simulink model "hybrid_new_eq_circuit_pascal5_single_shot_stack"  (R2019a)
settings: Solver=FixedStepAuto  StartTime=0.0  StopTime=sim_time  FixedStep=resolution  MinStep=0.001  RelTol=1e-4  EnableMultiTasking=on
values from neighbouring files (symbols this model uses):
  amps_in = double(amps_in)    [ClassHybrid.m]    (also in Sc.m = double(amps_in_); workspace_test_model.mat = 0)
  resolution = double(resolution)    [ClassHybrid.m]    (also in Sc.m = double(resolution_); matlab.mat = 1; model_out_all.mat = 0.5; testHyb.m = 0.5)
  tStep = resolution    (= 0.1)    [ClassHybrid.m]    (also in Sc.m; matlab.mat = 10; model_out_all.mat = 1; raw.mat = 1)
libraries: powerlib x525, simulink x9
(part 5 of 8)

== system hybrid_new_eq_circuit_pascal5_single_shot_stack/Battery 2/Subsystem/Subsystem3 ==
  note: Export user input data
  v_r_in : Inport
  v_cap_in : Inport  Port=2
  i_leak_in : Inport  Port=3
  p_chg_in : Inport  Port=4
  p_leak_in : Inport  Port=5
  i_in : Inport  Port=6
  c_in : Inport  Port=7
  r_in : Inport  Port=8
  r_leak_in : Inport  Port=9
  l_in : Inport  Port=10
  Constant : Constant  Value=c
  Constant4 : Constant  Value=r_esr
  Constant5 : Constant  Value=r_leak
  Fcn1 : Fcn  Expr=u^2/r_leak
  Mux{,1..9} (10 alike) : Mux  Inputs=2
  Parallel RLC Branch1 : powerlib/Elements/Parallel RLC Branch  LConnTagsString=a  RConnTagsString=__new0  BranchType=R  Resistance=r_leak  Inductance=1e-3  SetiL0=off  InitialCurrent=0  Capacitance=1e-6  Setx0=off  InitialVoltage=0  Measurements=None
      settings: SourceProductName=Simscape Electrical
  Parallel RLC Branch10 : powerlib/Elements/Parallel RLC Branch  LConnTagsString=a  RConnTagsString=__new0  BranchType=R  Resistance=r_esr  Inductance=1e-3  SetiL0=off  InitialCurrent=0  Capacitance=1e-6  Setx0=off  InitialVoltage=0  Measurements=None
      settings: SourceProductName=Simscape Electrical
  Parallel RLC Branch11 : powerlib/Elements/Parallel RLC Branch  LConnTagsString=a  RConnTagsString=__new0  BranchType=C  Resistance=1  Inductance=1e-3  SetiL0=off  InitialCurrent=0  Capacitance=c  Setx0=on  InitialVoltage=v_init  Measurements=None
      settings: SourceProductName=Simscape Electrical
  i : powerlib/Measurements/Current Measurement  PhasorSimulation=off  OutputType=Complex  PSBequivalent=0
      settings: SourceProductName=Simscape Electrical
  i_leak : powerlib/Measurements/Current Measurement  PhasorSimulation=off  OutputType=Complex  PSBequivalent=0
      settings: SourceProductName=Simscape Electrical
  v^2/R : Fcn  Expr=u^2/r_esr
  v_cap : powerlib/Measurements/Voltage Measurement  PhasorSimulation=off  OutputType=Magnitude  PSBequivalent=0
      settings: SourceProductName=Simscape Electrical
  v_r : powerlib/Measurements/Voltage Measurement  PhasorSimulation=off  OutputType=Complex  PSBequivalent=0
      settings: SourceProductName=Simscape Electrical
  VCC_in : PMIOPort  Side=Left
  VSS_in : PMIOPort  Port=2  Side=Left
  VCC_out : PMIOPort  Tag=PMCPort  Port=3  Side=Right
  VSS_out : PMIOPort  Tag=PMCPort  Port=4  Side=Right
  v_r_out : Outport
  v_cap_out : Outport  Port=2
  i_leak_out : Outport  Port=3
  p_chg_out : Outport  Port=4
  p_leak_out : Outport  Port=5
  i_out : Outport  Port=6
  c_out : Outport  Port=7
  r_out : Outport  Port=8
  r_leak_out : Outport  Port=9
  l_out : Outport  Port=10
  wires:
  i_leak/1 -> Mux2/1
  v_r/1 -> Mux1/1, v^2/R/1
  Mux6/1 -> c_out/1
  Mux7/1 -> r_out/1
  Mux8/1 -> r_leak_out/1
  Mux9/1 -> l_out/1
  Constant/1 -> Mux6/1
  Constant4/1 -> Mux7/1
  Constant5/1 -> Mux8/1
  ? -> Mux9/1
  c_in/1 -> Mux6/2
  l_in/1 -> Mux9/2
  r_leak_in/1 -> Mux8/2
  r_in/1 -> Mux7/2
  p_chg_in/1 -> Mux3/2
  Mux3/1 -> p_chg_out/1
  v_r_in/1 -> Mux1/2
  Mux1/1 -> v_r_out/1
  v^2/R/1 -> Mux3/1
  Mux2/1 -> i_leak_out/1
  i_leak_in/1 -> Mux2/2
  i/1 -> Mux5/1
  Mux5/1 -> i_out/1
  i_in/1 -> Mux5/2
  p_leak_in/1 -> Mux4/2
  Mux4/1 -> p_leak_out/1
  Mux/1 -> v_cap_out/1
  v_cap_in/1 -> Mux/2
  Fcn1/1 -> Mux4/1
  v_cap/1 -> Fcn1/1, Mux/1  "v_cap_out"
  connections:
  Parallel RLC Branch1/RConn1 -- i_leak/LConn1
  VSS_out/RConn1 -- VSS_in/RConn1 -- i_leak/RConn1 -- Parallel RLC Branch11/RConn1 -- v_cap/LConn2
  v_cap/LConn1 -- i/RConn1 -- Parallel RLC Branch11/LConn1 -- Parallel RLC Branch1/LConn1
  VCC_out/RConn1 -- v_r/LConn1 -- Parallel RLC Branch10/LConn1 -- VCC_in/RConn1
  v_r/LConn2 -- i/LConn1 -- Parallel RLC Branch10/RConn1

== system hybrid_new_eq_circuit_pascal5_single_shot_stack/Battery 2/Subsystem/Subsystem5 ==
  note: Export user input data
  v_r_in : Inport
  v_cap_in : Inport  Port=2
  i_leak_in : Inport  Port=3
  p_chg_in : Inport  Port=4
  p_leak_in : Inport  Port=5
  i_in : Inport  Port=6
  c_in : Inport  Port=7
  r_in : Inport  Port=8
  r_leak_in : Inport  Port=9
  l_in : Inport  Port=10
  Constant : Constant  Value=c
  Constant4 : Constant  Value=r_esr
  Constant5 : Constant  Value=r_leak
  Fcn1 : Fcn  Expr=u^2/r_leak
  Mux{,1..9} (10 alike) : Mux  Inputs=2
  Parallel RLC Branch1 : powerlib/Elements/Parallel RLC Branch  LConnTagsString=a  RConnTagsString=__new0  BranchType=R  Resistance=r_leak  Inductance=1e-3  SetiL0=off  InitialCurrent=0  Capacitance=1e-6  Setx0=off  InitialVoltage=0  Measurements=None
      settings: SourceProductName=Simscape Electrical
  Parallel RLC Branch10 : powerlib/Elements/Parallel RLC Branch  LConnTagsString=a  RConnTagsString=__new0  BranchType=R  Resistance=r_esr  Inductance=1e-3  SetiL0=off  InitialCurrent=0  Capacitance=1e-6  Setx0=off  InitialVoltage=0  Measurements=None
      settings: SourceProductName=Simscape Electrical
  Parallel RLC Branch11 : powerlib/Elements/Parallel RLC Branch  LConnTagsString=a  RConnTagsString=__new0  BranchType=C  Resistance=1  Inductance=1e-3  SetiL0=off  InitialCurrent=0  Capacitance=c  Setx0=on  InitialVoltage=v_init  Measurements=None
      settings: SourceProductName=Simscape Electrical
  i : powerlib/Measurements/Current Measurement  PhasorSimulation=off  OutputType=Complex  PSBequivalent=0
      settings: SourceProductName=Simscape Electrical
  i_leak : powerlib/Measurements/Current Measurement  PhasorSimulation=off  OutputType=Complex  PSBequivalent=0
      settings: SourceProductName=Simscape Electrical
  v^2/R : Fcn  Expr=u^2/r_esr
  v_cap : powerlib/Measurements/Voltage Measurement  PhasorSimulation=off  OutputType=Magnitude  PSBequivalent=0
      settings: SourceProductName=Simscape Electrical
  v_r : powerlib/Measurements/Voltage Measurement  PhasorSimulation=off  OutputType=Complex  PSBequivalent=0
      settings: SourceProductName=Simscape Electrical
  VCC_in : PMIOPort  Side=Left
  VSS_in : PMIOPort  Port=2  Side=Left
  VCC_out : PMIOPort  Tag=PMCPort  Port=3  Side=Right
  VSS_out : PMIOPort  Tag=PMCPort  Port=4  Side=Right
  v_r_out : Outport
  v_cap_out : Outport  Port=2
  i_leak_out : Outport  Port=3
  p_chg_out : Outport  Port=4
  p_leak_out : Outport  Port=5
  i_out : Outport  Port=6
  c_out : Outport  Port=7
  r_out : Outport  Port=8
  r_leak_out : Outport  Port=9
  l_out : Outport  Port=10
  wires:
  Fcn1/1 -> Mux4/1
  v_cap_in/1 -> Mux/2
  Mux/1 -> v_cap_out/1
  Mux4/1 -> p_leak_out/1
  p_leak_in/1 -> Mux4/2
  i_in/1 -> Mux5/2
  Mux5/1 -> i_out/1
  i/1 -> Mux5/1
  i_leak_in/1 -> Mux2/2
  Mux2/1 -> i_leak_out/1
  v^2/R/1 -> Mux3/1
  Mux1/1 -> v_r_out/1
  v_r_in/1 -> Mux1/2
  Mux3/1 -> p_chg_out/1
  p_chg_in/1 -> Mux3/2
  r_in/1 -> Mux7/2
  r_leak_in/1 -> Mux8/2
  l_in/1 -> Mux9/2
  c_in/1 -> Mux6/2
  ? -> Mux9/1
  Constant5/1 -> Mux8/1
  Constant4/1 -> Mux7/1
  Constant/1 -> Mux6/1
  Mux9/1 -> l_out/1
  Mux8/1 -> r_leak_out/1
  Mux7/1 -> r_out/1
  Mux6/1 -> c_out/1
  v_r/1 -> v^2/R/1, Mux1/1
  i_leak/1 -> Mux2/1
  v_cap/1 -> Fcn1/1, Mux/1  "v_cap_out"
  connections:
  Parallel RLC Branch10/RConn1 -- i/LConn1 -- v_r/LConn2
  VCC_in/RConn1 -- Parallel RLC Branch10/LConn1 -- v_r/LConn1 -- VCC_out/RConn1
  Parallel RLC Branch11/LConn1 -- i/RConn1 -- Parallel RLC Branch1/LConn1 -- v_cap/LConn1
  v_cap/LConn2 -- Parallel RLC Branch11/RConn1 -- i_leak/RConn1 -- VSS_in/RConn1 -- VSS_out/RConn1
  Parallel RLC Branch1/RConn1 -- i_leak/LConn1

== system hybrid_new_eq_circuit_pascal5_single_shot_stack/Battery 3/Subsystem/Subsystem1 ==
  note: Export user input data
  v_r_in : Inport
  v_cap_in : Inport  Port=2
  i_leak_in : Inport  Port=3
  p_chg_in : Inport  Port=4
  p_leak_in : Inport  Port=5
  i_in : Inport  Port=6
  c_in : Inport  Port=7
  r_in : Inport  Port=8
  r_leak_in : Inport  Port=9
  l_in : Inport  Port=10
  Constant : Constant  Value=c
  Constant4 : Constant  Value=r_esr
  Constant5 : Constant  Value=r_leak
  Fcn1 : Fcn  Expr=u^2/r_leak
  Mux{,1..9} (10 alike) : Mux  Inputs=2
  Parallel RLC Branch1 : powerlib/Elements/Parallel RLC Branch  LConnTagsString=a  RConnTagsString=__new0  BranchType=R  Resistance=r_leak  Inductance=1e-3  SetiL0=off  InitialCurrent=0  Capacitance=1e-6  Setx0=off  InitialVoltage=0  Measurements=None
      settings: SourceProductName=Simscape Electrical
  Parallel RLC Branch10 : powerlib/Elements/Parallel RLC Branch  LConnTagsString=a  RConnTagsString=__new0  BranchType=R  Resistance=r_esr  Inductance=1e-3  SetiL0=off  InitialCurrent=0  Capacitance=1e-6  Setx0=off  InitialVoltage=0  Measurements=None
      settings: SourceProductName=Simscape Electrical
  Parallel RLC Branch11 : powerlib/Elements/Parallel RLC Branch  LConnTagsString=a  RConnTagsString=__new0  BranchType=C  Resistance=1  Inductance=1e-3  SetiL0=off  InitialCurrent=0  Capacitance=c  Setx0=on  InitialVoltage=v_init  Measurements=None
      settings: SourceProductName=Simscape Electrical
  i : powerlib/Measurements/Current Measurement  PhasorSimulation=off  OutputType=Complex  PSBequivalent=0
      settings: SourceProductName=Simscape Electrical
  i_leak : powerlib/Measurements/Current Measurement  PhasorSimulation=off  OutputType=Complex  PSBequivalent=0
      settings: SourceProductName=Simscape Electrical
  v^2/R : Fcn  Expr=u^2/r_esr
  v_cap : powerlib/Measurements/Voltage Measurement  PhasorSimulation=off  OutputType=Magnitude  PSBequivalent=0
      settings: SourceProductName=Simscape Electrical
  v_r : powerlib/Measurements/Voltage Measurement  PhasorSimulation=off  OutputType=Complex  PSBequivalent=0
      settings: SourceProductName=Simscape Electrical
  VCC_in : PMIOPort  Side=Left
  VSS_in : PMIOPort  Port=2  Side=Left
  VCC_out : PMIOPort  Tag=PMCPort  Port=3  Side=Right
  VSS_out : PMIOPort  Tag=PMCPort  Port=4  Side=Right
  v_r_out : Outport
  v_cap_out : Outport  Port=2
  i_leak_out : Outport  Port=3
  p_chg_out : Outport  Port=4
  p_leak_out : Outport  Port=5
  i_out : Outport  Port=6
  c_out : Outport  Port=7
  r_out : Outport  Port=8
  r_leak_out : Outport  Port=9
  l_out : Outport  Port=10
  wires:
  i_leak/1 -> Mux2/1
  v_r/1 -> Mux1/1, v^2/R/1
  Mux6/1 -> c_out/1
  Mux7/1 -> r_out/1
  Mux8/1 -> r_leak_out/1
  Mux9/1 -> l_out/1
  Constant/1 -> Mux6/1
  Constant4/1 -> Mux7/1
  Constant5/1 -> Mux8/1
  ? -> Mux9/1
  c_in/1 -> Mux6/2
  l_in/1 -> Mux9/2
  r_leak_in/1 -> Mux8/2
  r_in/1 -> Mux7/2
  p_chg_in/1 -> Mux3/2
  Mux3/1 -> p_chg_out/1
  v_r_in/1 -> Mux1/2
  Mux1/1 -> v_r_out/1
  v^2/R/1 -> Mux3/1
  Mux2/1 -> i_leak_out/1
  i_leak_in/1 -> Mux2/2
  i/1 -> Mux5/1
  Mux5/1 -> i_out/1
  i_in/1 -> Mux5/2
  p_leak_in/1 -> Mux4/2
  Mux4/1 -> p_leak_out/1
  Mux/1 -> v_cap_out/1
  v_cap_in/1 -> Mux/2
  Fcn1/1 -> Mux4/1
  v_cap/1 -> Fcn1/1, Mux/1  "v_cap_out"
  connections:
  Parallel RLC Branch1/RConn1 -- i_leak/LConn1
  VSS_out/RConn1 -- VSS_in/RConn1 -- i_leak/RConn1 -- Parallel RLC Branch11/RConn1 -- v_cap/LConn2
  v_cap/LConn1 -- i/RConn1 -- Parallel RLC Branch11/LConn1 -- Parallel RLC Branch1/LConn1
  VCC_out/RConn1 -- v_r/LConn1 -- Parallel RLC Branch10/LConn1 -- VCC_in/RConn1
  v_r/LConn2 -- i/LConn1 -- Parallel RLC Branch10/RConn1

== system hybrid_new_eq_circuit_pascal5_single_shot_stack/Battery 3/Subsystem/Subsystem2 ==
  note: Export user input data
  v_r_in : Inport
  v_cap_in : Inport  Port=2
  i_leak_in : Inport  Port=3
  p_chg_in : Inport  Port=4
  p_leak_in : Inport  Port=5
  i_in : Inport  Port=6
  c_in : Inport  Port=7
  r_in : Inport  Port=8
  r_leak_in : Inport  Port=9
  l_in : Inport  Port=10
  Constant : Constant  Value=c
  Constant4 : Constant  Value=r_esr
  Constant5 : Constant  Value=r_leak
  Fcn1 : Fcn  Expr=u^2/r_leak
  Mux{,1..9} (10 alike) : Mux  Inputs=2
  Parallel RLC Branch1 : powerlib/Elements/Parallel RLC Branch  LConnTagsString=a  RConnTagsString=__new0  BranchType=R  Resistance=r_leak  Inductance=1e-3  SetiL0=off  InitialCurrent=0  Capacitance=1e-6  Setx0=off  InitialVoltage=0  Measurements=None
      settings: SourceProductName=Simscape Electrical
  Parallel RLC Branch10 : powerlib/Elements/Parallel RLC Branch  LConnTagsString=a  RConnTagsString=__new0  BranchType=R  Resistance=r_esr  Inductance=1e-3  SetiL0=off  InitialCurrent=0  Capacitance=1e-6  Setx0=off  InitialVoltage=0  Measurements=None
      settings: SourceProductName=Simscape Electrical
  Parallel RLC Branch11 : powerlib/Elements/Parallel RLC Branch  LConnTagsString=a  RConnTagsString=__new0  BranchType=C  Resistance=1  Inductance=1e-3  SetiL0=off  InitialCurrent=0  Capacitance=c  Setx0=on  InitialVoltage=v_init  Measurements=None
      settings: SourceProductName=Simscape Electrical
  i : powerlib/Measurements/Current Measurement  PhasorSimulation=off  OutputType=Complex  PSBequivalent=0
      settings: SourceProductName=Simscape Electrical
  i_leak : powerlib/Measurements/Current Measurement  PhasorSimulation=off  OutputType=Complex  PSBequivalent=0
      settings: SourceProductName=Simscape Electrical
  v^2/R : Fcn  Expr=u^2/r_esr
  v_cap : powerlib/Measurements/Voltage Measurement  PhasorSimulation=off  OutputType=Magnitude  PSBequivalent=0
      settings: SourceProductName=Simscape Electrical
  v_r : powerlib/Measurements/Voltage Measurement  PhasorSimulation=off  OutputType=Complex  PSBequivalent=0
      settings: SourceProductName=Simscape Electrical
  VCC_in : PMIOPort  Side=Left
  VSS_in : PMIOPort  Port=2  Side=Left
  VCC_out : PMIOPort  Tag=PMCPort  Port=3  Side=Right
  VSS_out : PMIOPort  Tag=PMCPort  Port=4  Side=Right
  v_r_out : Outport
  v_cap_out : Outport  Port=2
  i_leak_out : Outport  Port=3
  p_chg_out : Outport  Port=4
  p_leak_out : Outport  Port=5
  i_out : Outport  Port=6
  c_out : Outport  Port=7
  r_out : Outport  Port=8
  r_leak_out : Outport  Port=9
  l_out : Outport  Port=10
  wires:
  Fcn1/1 -> Mux4/1
  v_cap_in/1 -> Mux/2
  Mux/1 -> v_cap_out/1
  Mux4/1 -> p_leak_out/1
  p_leak_in/1 -> Mux4/2
  i_in/1 -> Mux5/2
  Mux5/1 -> i_out/1
  i/1 -> Mux5/1
  i_leak_in/1 -> Mux2/2
  Mux2/1 -> i_leak_out/1
  v^2/R/1 -> Mux3/1
  Mux1/1 -> v_r_out/1
  v_r_in/1 -> Mux1/2
  Mux3/1 -> p_chg_out/1
  p_chg_in/1 -> Mux3/2
  r_in/1 -> Mux7/2
  r_leak_in/1 -> Mux8/2
  l_in/1 -> Mux9/2
  c_in/1 -> Mux6/2
  ? -> Mux9/1
  Constant5/1 -> Mux8/1
  Constant4/1 -> Mux7/1
  Constant/1 -> Mux6/1
  Mux9/1 -> l_out/1
  Mux8/1 -> r_leak_out/1
  Mux7/1 -> r_out/1
  Mux6/1 -> c_out/1
  v_r/1 -> v^2/R/1, Mux1/1
  i_leak/1 -> Mux2/1
  v_cap/1 -> Mux/1, Fcn1/1  "v_cap_out"
  connections:
  Parallel RLC Branch10/RConn1 -- i/LConn1 -- v_r/LConn2
  VCC_in/RConn1 -- Parallel RLC Branch10/LConn1 -- v_r/LConn1 -- VCC_out/RConn1
  Parallel RLC Branch1/LConn1 -- Parallel RLC Branch11/LConn1 -- i/RConn1 -- v_cap/LConn1
  v_cap/LConn2 -- Parallel RLC Branch11/RConn1 -- i_leak/RConn1 -- VSS_in/RConn1 -- VSS_out/RConn1
  Parallel RLC Branch1/RConn1 -- i_leak/LConn1

== system hybrid_new_eq_circuit_pascal5_single_shot_stack/Battery 3/Subsystem/Subsystem3 ==
  note: Export user input data
  v_r_in : Inport
  v_cap_in : Inport  Port=2
  i_leak_in : Inport  Port=3
  p_chg_in : Inport  Port=4
  p_leak_in : Inport  Port=5
  i_in : Inport  Port=6
  c_in : Inport  Port=7
  r_in : Inport  Port=8
  r_leak_in : Inport  Port=9
  l_in : Inport  Port=10
  Constant : Constant  Value=c
  Constant4 : Constant  Value=r_esr
  Constant5 : Constant  Value=r_leak
  Fcn1 : Fcn  Expr=u^2/r_leak
  Mux{,1..9} (10 alike) : Mux  Inputs=2
  Parallel RLC Branch1 : powerlib/Elements/Parallel RLC Branch  LConnTagsString=a  RConnTagsString=__new0  BranchType=R  Resistance=r_leak  Inductance=1e-3  SetiL0=off  InitialCurrent=0  Capacitance=1e-6  Setx0=off  InitialVoltage=0  Measurements=None
      settings: SourceProductName=Simscape Electrical
  Parallel RLC Branch10 : powerlib/Elements/Parallel RLC Branch  LConnTagsString=a  RConnTagsString=__new0  BranchType=R  Resistance=r_esr  Inductance=1e-3  SetiL0=off  InitialCurrent=0  Capacitance=1e-6  Setx0=off  InitialVoltage=0  Measurements=None
      settings: SourceProductName=Simscape Electrical
  Parallel RLC Branch11 : powerlib/Elements/Parallel RLC Branch  LConnTagsString=a  RConnTagsString=__new0  BranchType=C  Resistance=1  Inductance=1e-3  SetiL0=off  InitialCurrent=0  Capacitance=c  Setx0=on  InitialVoltage=v_init  Measurements=None
      settings: SourceProductName=Simscape Electrical
  i : powerlib/Measurements/Current Measurement  PhasorSimulation=off  OutputType=Complex  PSBequivalent=0
      settings: SourceProductName=Simscape Electrical
  i_leak : powerlib/Measurements/Current Measurement  PhasorSimulation=off  OutputType=Complex  PSBequivalent=0
      settings: SourceProductName=Simscape Electrical
  v^2/R : Fcn  Expr=u^2/r_esr
  v_cap : powerlib/Measurements/Voltage Measurement  PhasorSimulation=off  OutputType=Magnitude  PSBequivalent=0
      settings: SourceProductName=Simscape Electrical
  v_r : powerlib/Measurements/Voltage Measurement  PhasorSimulation=off  OutputType=Complex  PSBequivalent=0
      settings: SourceProductName=Simscape Electrical
  VCC_in : PMIOPort  Side=Left
  VSS_in : PMIOPort  Port=2  Side=Left
  VCC_out : PMIOPort  Tag=PMCPort  Port=3  Side=Right
  VSS_out : PMIOPort  Tag=PMCPort  Port=4  Side=Right
  v_r_out : Outport
  v_cap_out : Outport  Port=2
  i_leak_out : Outport  Port=3
  p_chg_out : Outport  Port=4
  p_leak_out : Outport  Port=5
  i_out : Outport  Port=6
  c_out : Outport  Port=7
  r_out : Outport  Port=8
  r_leak_out : Outport  Port=9
  l_out : Outport  Port=10
  wires:
  i_leak/1 -> Mux2/1
  v_r/1 -> Mux1/1, v^2/R/1
  Mux6/1 -> c_out/1
  Mux7/1 -> r_out/1
  Mux8/1 -> r_leak_out/1
  Mux9/1 -> l_out/1
  Constant/1 -> Mux6/1
  Constant4/1 -> Mux7/1
  Constant5/1 -> Mux8/1
  ? -> Mux9/1
  c_in/1 -> Mux6/2
  l_in/1 -> Mux9/2
  r_leak_in/1 -> Mux8/2
  r_in/1 -> Mux7/2
  p_chg_in/1 -> Mux3/2
  Mux3/1 -> p_chg_out/1
  v_r_in/1 -> Mux1/2
  Mux1/1 -> v_r_out/1
  v^2/R/1 -> Mux3/1
  Mux2/1 -> i_leak_out/1
  i_leak_in/1 -> Mux2/2
  i/1 -> Mux5/1
  Mux5/1 -> i_out/1
  i_in/1 -> Mux5/2
  p_leak_in/1 -> Mux4/2
  Mux4/1 -> p_leak_out/1
  Mux/1 -> v_cap_out/1
  v_cap_in/1 -> Mux/2
  Fcn1/1 -> Mux4/1
  v_cap/1 -> Fcn1/1, Mux/1  "v_cap_out"
  connections:
  Parallel RLC Branch1/RConn1 -- i_leak/LConn1
  VSS_out/RConn1 -- VSS_in/RConn1 -- i_leak/RConn1 -- Parallel RLC Branch11/RConn1 -- v_cap/LConn2
  v_cap/LConn1 -- i/RConn1 -- Parallel RLC Branch11/LConn1 -- Parallel RLC Branch1/LConn1
  VCC_out/RConn1 -- v_r/LConn1 -- Parallel RLC Branch10/LConn1 -- VCC_in/RConn1
  v_r/LConn2 -- i/LConn1 -- Parallel RLC Branch10/RConn1

== system hybrid_new_eq_circuit_pascal5_single_shot_stack/Battery 3/Subsystem/Subsystem5 ==
  note: Export user input data
  v_r_in : Inport
  v_cap_in : Inport  Port=2
  i_leak_in : Inport  Port=3
  p_chg_in : Inport  Port=4
  p_leak_in : Inport  Port=5
  i_in : Inport  Port=6
  c_in : Inport  Port=7
  r_in : Inport  Port=8
  r_leak_in : Inport  Port=9
  l_in : Inport  Port=10
  Constant : Constant  Value=c
  Constant4 : Constant  Value=r_esr
  Constant5 : Constant  Value=r_leak
  Fcn1 : Fcn  Expr=u^2/r_leak
  Mux{,1..9} (10 alike) : Mux  Inputs=2
  Parallel RLC Branch1 : powerlib/Elements/Parallel RLC Branch  LConnTagsString=a  RConnTagsString=__new0  BranchType=R  Resistance=r_leak  Inductance=1e-3  SetiL0=off  InitialCurrent=0  Capacitance=1e-6  Setx0=off  InitialVoltage=0  Measurements=None
      settings: SourceProductName=Simscape Electrical
  Parallel RLC Branch10 : powerlib/Elements/Parallel RLC Branch  LConnTagsString=a  RConnTagsString=__new0  BranchType=R  Resistance=r_esr  Inductance=1e-3  SetiL0=off  InitialCurrent=0  Capacitance=1e-6  Setx0=off  InitialVoltage=0  Measurements=None
      settings: SourceProductName=Simscape Electrical
  Parallel RLC Branch11 : powerlib/Elements/Parallel RLC Branch  LConnTagsString=a  RConnTagsString=__new0  BranchType=C  Resistance=1  Inductance=1e-3  SetiL0=off  InitialCurrent=0  Capacitance=c  Setx0=on  InitialVoltage=v_init  Measurements=None
      settings: SourceProductName=Simscape Electrical
  i : powerlib/Measurements/Current Measurement  PhasorSimulation=off  OutputType=Complex  PSBequivalent=0
      settings: SourceProductName=Simscape Electrical
  i_leak : powerlib/Measurements/Current Measurement  PhasorSimulation=off  OutputType=Complex  PSBequivalent=0
      settings: SourceProductName=Simscape Electrical
  v^2/R : Fcn  Expr=u^2/r_esr
  v_cap : powerlib/Measurements/Voltage Measurement  PhasorSimulation=off  OutputType=Magnitude  PSBequivalent=0
      settings: SourceProductName=Simscape Electrical
  v_r : powerlib/Measurements/Voltage Measurement  PhasorSimulation=off  OutputType=Complex  PSBequivalent=0
      settings: SourceProductName=Simscape Electrical
  VCC_in : PMIOPort  Side=Left
  VSS_in : PMIOPort  Port=2  Side=Left
  VCC_out : PMIOPort  Tag=PMCPort  Port=3  Side=Right
  VSS_out : PMIOPort  Tag=PMCPort  Port=4  Side=Right
  v_r_out : Outport
  v_cap_out : Outport  Port=2
  i_leak_out : Outport  Port=3
  p_chg_out : Outport  Port=4
  p_leak_out : Outport  Port=5
  i_out : Outport  Port=6
  c_out : Outport  Port=7
  r_out : Outport  Port=8
  r_leak_out : Outport  Port=9
  l_out : Outport  Port=10
  wires:
  Fcn1/1 -> Mux4/1
  v_cap_in/1 -> Mux/2
  Mux/1 -> v_cap_out/1
  Mux4/1 -> p_leak_out/1
  p_leak_in/1 -> Mux4/2
  i_in/1 -> Mux5/2
  Mux5/1 -> i_out/1
  i/1 -> Mux5/1
  i_leak_in/1 -> Mux2/2
  Mux2/1 -> i_leak_out/1
  v^2/R/1 -> Mux3/1
  Mux1/1 -> v_r_out/1
  v_r_in/1 -> Mux1/2
  Mux3/1 -> p_chg_out/1
  p_chg_in/1 -> Mux3/2
  r_in/1 -> Mux7/2
  r_leak_in/1 -> Mux8/2
  l_in/1 -> Mux9/2
  c_in/1 -> Mux6/2
  ? -> Mux9/1
  Constant5/1 -> Mux8/1
  Constant4/1 -> Mux7/1
  Constant/1 -> Mux6/1
  Mux9/1 -> l_out/1
  Mux8/1 -> r_leak_out/1
  Mux7/1 -> r_out/1
  Mux6/1 -> c_out/1
  v_r/1 -> v^2/R/1, Mux1/1
  i_leak/1 -> Mux2/1
  v_cap/1 -> Fcn1/1, Mux/1  "v_cap_out"
  connections:
  Parallel RLC Branch10/RConn1 -- i/LConn1 -- v_r/LConn2
  VCC_in/RConn1 -- Parallel RLC Branch10/LConn1 -- v_r/LConn1 -- VCC_out/RConn1
  Parallel RLC Branch11/LConn1 -- i/RConn1 -- Parallel RLC Branch1/LConn1 -- v_cap/LConn1
  v_cap/LConn2 -- Parallel RLC Branch11/RConn1 -- i_leak/RConn1 -- VSS_in/RConn1 -- VSS_out/RConn1
  Parallel RLC Branch1/RConn1 -- i_leak/LConn1

== system hybrid_new_eq_circuit_pascal5_single_shot_stack/Supercapacitor 1/Subsystem/Subsystem1 ==
  note: Export user input data
  v_r_in : Inport
  v_cap_in : Inport  Port=2
  i_leak_in : Inport  Port=3
  p_chg_in : Inport  Port=4
  p_leak_in : Inport  Port=5
  i_in : Inport  Port=6
  c_in : Inport  Port=7
  r_in : Inport  Port=8
  r_leak_in : Inport  Port=9
  l_in : Inport  Port=10
  Constant : Constant  Value=c
  Constant4 : Constant  Value=r_esr
  Constant5 : Constant  Value=r_leak
  Fcn1 : Fcn  Expr=u^2/r_leak
  Mux{,1..9} (10 alike) : Mux  Inputs=2
  Parallel RLC Branch1 : powerlib/Elements/Parallel RLC Branch  LConnTagsString=a  RConnTagsString=__new0  BranchType=R  Resistance=r_leak  Inductance=1e-3  SetiL0=off  InitialCurrent=0  Capacitance=1e-6  Setx0=off  InitialVoltage=0  Measurements=None
      settings: SourceProductName=Simscape Electrical
  Parallel RLC Branch10 : powerlib/Elements/Parallel RLC Branch  LConnTagsString=a  RConnTagsString=__new0  BranchType=R  Resistance=r_esr  Inductance=1e-3  SetiL0=off  InitialCurrent=0  Capacitance=1e-6  Setx0=off  InitialVoltage=0  Measurements=None
      settings: SourceProductName=Simscape Electrical
  Parallel RLC Branch11 : powerlib/Elements/Parallel RLC Branch  LConnTagsString=a  RConnTagsString=__new0  BranchType=C  Resistance=1  Inductance=1e-3  SetiL0=off  InitialCurrent=0  Capacitance=c  Setx0=on  InitialVoltage=v_init  Measurements=None
      settings: SourceProductName=Simscape Electrical
  i : powerlib/Measurements/Current Measurement  PhasorSimulation=off  OutputType=Complex  PSBequivalent=0
      settings: SourceProductName=Simscape Electrical
  i_leak : powerlib/Measurements/Current Measurement  PhasorSimulation=off  OutputType=Complex  PSBequivalent=0
      settings: SourceProductName=Simscape Electrical
  v^2/R : Fcn  Expr=u^2/r_esr
  v_cap : powerlib/Measurements/Voltage Measurement  PhasorSimulation=off  OutputType=Complex  PSBequivalent=0
      settings: SourceProductName=Simscape Electrical
  v_r : powerlib/Measurements/Voltage Measurement  PhasorSimulation=off  OutputType=Complex  PSBequivalent=0
      settings: SourceProductName=Simscape Electrical
  VCC_in : PMIOPort  Side=Left
  VSS_in : PMIOPort  Port=2  Side=Left
  VCC_out : PMIOPort  Tag=PMCPort  Port=3  Side=Right
  VSS_out : PMIOPort  Tag=PMCPort  Port=4  Side=Right
  v_r_out : Outport
  v_cap_out : Outport  Port=2
  i_leak_out : Outport  Port=3
  p_chg_out : Outport  Port=4
  p_leak_out : Outport  Port=5
  i_out : Outport  Port=6
  c_out : Outport  Port=7
  r_out : Outport  Port=8
  r_leak_out : Outport  Port=9
  l_out : Outport  Port=10
  wires:
  Fcn1/1 -> Mux4/1
  v_cap/1 -> Mux/1, Fcn1/1
  v_cap_in/1 -> Mux/2
  Mux/1 -> v_cap_out/1
  Mux4/1 -> p_leak_out/1
  p_leak_in/1 -> Mux4/2
  i_in/1 -> Mux5/2
  Mux5/1 -> i_out/1
  i/1 -> Mux5/1
  i_leak_in/1 -> Mux2/2
  Mux2/1 -> i_leak_out/1
  v^2/R/1 -> Mux3/1
  Mux1/1 -> v_r_out/1
  v_r_in/1 -> Mux1/2
  Mux3/1 -> p_chg_out/1
  p_chg_in/1 -> Mux3/2
  r_in/1 -> Mux7/2
  r_leak_in/1 -> Mux8/2
  l_in/1 -> Mux9/2
  c_in/1 -> Mux6/2
  ? -> Mux9/1
  Constant5/1 -> Mux8/1
  Constant4/1 -> Mux7/1
  Constant/1 -> Mux6/1
  Mux9/1 -> l_out/1
  Mux8/1 -> r_leak_out/1
  Mux7/1 -> r_out/1
  Mux6/1 -> c_out/1
  v_r/1 -> v^2/R/1, Mux1/1
  i_leak/1 -> Mux2/1
  connections:
  Parallel RLC Branch10/RConn1 -- i/LConn1 -- v_r/LConn2
  VCC_in/RConn1 -- Parallel RLC Branch10/LConn1 -- v_r/LConn1 -- VCC_out/RConn1
  Parallel RLC Branch1/LConn1 -- Parallel RLC Branch11/LConn1 -- i/RConn1 -- v_cap/LConn1
  v_cap/LConn2 -- Parallel RLC Branch11/RConn1 -- i_leak/RConn1 -- VSS_in/RConn1 -- VSS_out/RConn1
  Parallel RLC Branch1/RConn1 -- i_leak/LConn1

== system hybrid_new_eq_circuit_pascal5_single_shot_stack/Supercapacitor 1/Subsystem/Subsystem2 ==
  note: Export user input data
  v_r_in : Inport
  v_cap_in : Inport  Port=2
  i_leak_in : Inport  Port=3
  p_chg_in : Inport  Port=4
  p_leak_in : Inport  Port=5
  i_in : Inport  Port=6
  c_in : Inport  Port=7
  r_in : Inport  Port=8
  r_leak_in : Inport  Port=9
  l_in : Inport  Port=10
  Constant : Constant  Value=c
  Constant4 : Constant  Value=r_esr
  Constant5 : Constant  Value=r_leak
  Fcn1 : Fcn  Expr=u^2/r_leak
  Mux{,1..9} (10 alike) : Mux  Inputs=2
  Parallel RLC Branch1 : powerlib/Elements/Parallel RLC Branch  LConnTagsString=a  RConnTagsString=__new0  BranchType=R  Resistance=r_leak  Inductance=1e-3  SetiL0=off  InitialCurrent=0  Capacitance=1e-6  Setx0=off  InitialVoltage=0  Measurements=None
      settings: SourceProductName=Simscape Electrical
  Parallel RLC Branch10 : powerlib/Elements/Parallel RLC Branch  LConnTagsString=a  RConnTagsString=__new0  BranchType=R  Resistance=r_esr  Inductance=1e-3  SetiL0=off  InitialCurrent=0  Capacitance=1e-6  Setx0=off  InitialVoltage=0  Measurements=None
      settings: SourceProductName=Simscape Electrical
  Parallel RLC Branch11 : powerlib/Elements/Parallel RLC Branch  LConnTagsString=a  RConnTagsString=__new0  BranchType=C  Resistance=1  Inductance=1e-3  SetiL0=off  InitialCurrent=0  Capacitance=c  Setx0=on  InitialVoltage=v_init  Measurements=None
      settings: SourceProductName=Simscape Electrical
  i : powerlib/Measurements/Current Measurement  PhasorSimulation=off  OutputType=Complex  PSBequivalent=0
      settings: SourceProductName=Simscape Electrical
  i_leak : powerlib/Measurements/Current Measurement  PhasorSimulation=off  OutputType=Complex  PSBequivalent=0
      settings: SourceProductName=Simscape Electrical
  v^2/R : Fcn  Expr=u^2/r_esr
  v_cap : powerlib/Measurements/Voltage Measurement  PhasorSimulation=off  OutputType=Complex  PSBequivalent=0
      settings: SourceProductName=Simscape Electrical
  v_r : powerlib/Measurements/Voltage Measurement  PhasorSimulation=off  OutputType=Complex  PSBequivalent=0
      settings: SourceProductName=Simscape Electrical
  VCC_in : PMIOPort  Side=Left
  VSS_in : PMIOPort  Port=2  Side=Left
  VCC_out : PMIOPort  Tag=PMCPort  Port=3  Side=Right
  VSS_out : PMIOPort  Tag=PMCPort  Port=4  Side=Right
  v_r_out : Outport
  v_cap_out : Outport  Port=2
  i_leak_out : Outport  Port=3
  p_chg_out : Outport  Port=4
  p_leak_out : Outport  Port=5
  i_out : Outport  Port=6
  c_out : Outport  Port=7
  r_out : Outport  Port=8
  r_leak_out : Outport  Port=9
  l_out : Outport  Port=10
  wires:
  i_leak/1 -> Mux2/1
  v_r/1 -> Mux1/1, v^2/R/1
  Mux6/1 -> c_out/1
  Mux7/1 -> r_out/1
  Mux8/1 -> r_leak_out/1
  Mux9/1 -> l_out/1
  Constant/1 -> Mux6/1
  Constant4/1 -> Mux7/1
  Constant5/1 -> Mux8/1
  ? -> Mux9/1
  c_in/1 -> Mux6/2
  l_in/1 -> Mux9/2
  r_leak_in/1 -> Mux8/2
  r_in/1 -> Mux7/2
  p_chg_in/1 -> Mux3/2
  Mux3/1 -> p_chg_out/1
  v_r_in/1 -> Mux1/2
  Mux1/1 -> v_r_out/1
  v^2/R/1 -> Mux3/1
  Mux2/1 -> i_leak_out/1
  i_leak_in/1 -> Mux2/2
  i/1 -> Mux5/1
  Mux5/1 -> i_out/1
  i_in/1 -> Mux5/2
  p_leak_in/1 -> Mux4/2
  Mux4/1 -> p_leak_out/1
  Mux/1 -> v_cap_out/1
  v_cap_in/1 -> Mux/2
  v_cap/1 -> Fcn1/1, Mux/1
  Fcn1/1 -> Mux4/1
  connections:
  Parallel RLC Branch1/RConn1 -- i_leak/LConn1
  VSS_out/RConn1 -- VSS_in/RConn1 -- i_leak/RConn1 -- Parallel RLC Branch11/RConn1 -- v_cap/LConn2
  v_cap/LConn1 -- i/RConn1 -- Parallel RLC Branch11/LConn1 -- Parallel RLC Branch1/LConn1
  VCC_out/RConn1 -- v_r/LConn1 -- Parallel RLC Branch10/LConn1 -- VCC_in/RConn1
  v_r/LConn2 -- i/LConn1 -- Parallel RLC Branch10/RConn1

== system hybrid_new_eq_circuit_pascal5_single_shot_stack/Supercapacitor 1/Subsystem/Subsystem3 ==
  note: Export user input data
  v_r_in : Inport
  v_cap_in : Inport  Port=2
  i_leak_in : Inport  Port=3
  p_chg_in : Inport  Port=4
  p_leak_in : Inport  Port=5
  i_in : Inport  Port=6
  c_in : Inport  Port=7
  r_in : Inport  Port=8
  r_leak_in : Inport  Port=9
  l_in : Inport  Port=10
  Constant : Constant  Value=c
  Constant4 : Constant  Value=r_esr
  Constant5 : Constant  Value=r_leak
  Fcn1 : Fcn  Expr=u^2/r_leak
  Mux{,1..9} (10 alike) : Mux  Inputs=2
  Parallel RLC Branch1 : powerlib/Elements/Parallel RLC Branch  LConnTagsString=a  RConnTagsString=__new0  BranchType=R  Resistance=r_leak  Inductance=1e-3  SetiL0=off  InitialCurrent=0  Capacitance=1e-6  Setx0=off  InitialVoltage=0  Measurements=None
      settings: SourceProductName=Simscape Electrical
  Parallel RLC Branch10 : powerlib/Elements/Parallel RLC Branch  LConnTagsString=a  RConnTagsString=__new0  BranchType=R  Resistance=r_esr  Inductance=1e-3  SetiL0=off  InitialCurrent=0  Capacitance=1e-6  Setx0=off  InitialVoltage=0  Measurements=None
      settings: SourceProductName=Simscape Electrical
  Parallel RLC Branch11 : powerlib/Elements/Parallel RLC Branch  LConnTagsString=a  RConnTagsString=__new0  BranchType=C  Resistance=1  Inductance=1e-3  SetiL0=off  InitialCurrent=0  Capacitance=c  Setx0=on  InitialVoltage=v_init  Measurements=None
      settings: SourceProductName=Simscape Electrical
  i : powerlib/Measurements/Current Measurement  PhasorSimulation=off  OutputType=Complex  PSBequivalent=0
      settings: SourceProductName=Simscape Electrical
  i_leak : powerlib/Measurements/Current Measurement  PhasorSimulation=off  OutputType=Complex  PSBequivalent=0
      settings: SourceProductName=Simscape Electrical
  v^2/R : Fcn  Expr=u^2/r_esr
  v_cap : powerlib/Measurements/Voltage Measurement  PhasorSimulation=off  OutputType=Complex  PSBequivalent=0
      settings: SourceProductName=Simscape Electrical
  v_r : powerlib/Measurements/Voltage Measurement  PhasorSimulation=off  OutputType=Complex  PSBequivalent=0
      settings: SourceProductName=Simscape Electrical
  VCC_in : PMIOPort  Side=Left
  VSS_in : PMIOPort  Port=2  Side=Left
  VCC_out : PMIOPort  Tag=PMCPort  Port=3  Side=Right
  VSS_out : PMIOPort  Tag=PMCPort  Port=4  Side=Right
  v_r_out : Outport
  v_cap_out : Outport  Port=2
  i_leak_out : Outport  Port=3
  p_chg_out : Outport  Port=4
  p_leak_out : Outport  Port=5
  i_out : Outport  Port=6
  c_out : Outport  Port=7
  r_out : Outport  Port=8
  r_leak_out : Outport  Port=9
  l_out : Outport  Port=10
  wires:
  Fcn1/1 -> Mux4/1
  v_cap/1 -> Mux/1, Fcn1/1
  v_cap_in/1 -> Mux/2
  Mux/1 -> v_cap_out/1
  Mux4/1 -> p_leak_out/1
  p_leak_in/1 -> Mux4/2
  i_in/1 -> Mux5/2
  Mux5/1 -> i_out/1
  i/1 -> Mux5/1
  i_leak_in/1 -> Mux2/2
  Mux2/1 -> i_leak_out/1
  v^2/R/1 -> Mux3/1
  Mux1/1 -> v_r_out/1
  v_r_in/1 -> Mux1/2
  Mux3/1 -> p_chg_out/1
  p_chg_in/1 -> Mux3/2
  r_in/1 -> Mux7/2
  r_leak_in/1 -> Mux8/2
  l_in/1 -> Mux9/2
  c_in/1 -> Mux6/2
  ? -> Mux9/1
  Constant5/1 -> Mux8/1
  Constant4/1 -> Mux7/1
  Constant/1 -> Mux6/1
  Mux9/1 -> l_out/1
  Mux8/1 -> r_leak_out/1
  Mux7/1 -> r_out/1
  Mux6/1 -> c_out/1
  v_r/1 -> v^2/R/1, Mux1/1
  i_leak/1 -> Mux2/1
  connections:
  Parallel RLC Branch10/RConn1 -- i/LConn1 -- v_r/LConn2
  VCC_in/RConn1 -- Parallel RLC Branch10/LConn1 -- v_r/LConn1 -- VCC_out/RConn1
  Parallel RLC Branch1/LConn1 -- Parallel RLC Branch11/LConn1 -- i/RConn1 -- v_cap/LConn1
  v_cap/LConn2 -- Parallel RLC Branch11/RConn1 -- i_leak/RConn1 -- VSS_in/RConn1 -- VSS_out/RConn1
  Parallel RLC Branch1/RConn1 -- i_leak/LConn1

== system hybrid_new_eq_circuit_pascal5_single_shot_stack/Supercapacitor 1/Subsystem/Subsystem5 ==
  note: Export user input data
  v_r_in : Inport
  v_cap_in : Inport  Port=2
  i_leak_in : Inport  Port=3
  p_chg_in : Inport  Port=4
  p_leak_in : Inport  Port=5
  i_in : Inport  Port=6
  c_in : Inport  Port=7
  r_in : Inport  Port=8
  r_leak_in : Inport  Port=9
  l_in : Inport  Port=10
  Constant : Constant  Value=c
  Constant4 : Constant  Value=r_esr
  Constant5 : Constant  Value=r_leak
  Fcn1 : Fcn  Expr=u^2/r_leak
  Mux{,1..9} (10 alike) : Mux  Inputs=2
  Parallel RLC Branch1 : powerlib/Elements/Parallel RLC Branch  LConnTagsString=a  RConnTagsString=__new0  BranchType=R  Resistance=r_leak  Inductance=1e-3  SetiL0=off  InitialCurrent=0  Capacitance=1e-6  Setx0=off  InitialVoltage=0  Measurements=None
      settings: SourceProductName=Simscape Electrical
  Parallel RLC Branch10 : powerlib/Elements/Parallel RLC Branch  LConnTagsString=a  RConnTagsString=__new0  BranchType=R  Resistance=r_esr  Inductance=1e-3  SetiL0=off  InitialCurrent=0  Capacitance=1e-6  Setx0=off  InitialVoltage=0  Measurements=None
      settings: SourceProductName=Simscape Electrical
  Parallel RLC Branch11 : powerlib/Elements/Parallel RLC Branch  LConnTagsString=a  RConnTagsString=__new0  BranchType=C  Resistance=1  Inductance=1e-3  SetiL0=off  InitialCurrent=0  Capacitance=c  Setx0=on  InitialVoltage=v_init  Measurements=None
      settings: SourceProductName=Simscape Electrical
  i : powerlib/Measurements/Current Measurement  PhasorSimulation=off  OutputType=Complex  PSBequivalent=0
      settings: SourceProductName=Simscape Electrical
  i_leak : powerlib/Measurements/Current Measurement  PhasorSimulation=off  OutputType=Complex  PSBequivalent=0
      settings: SourceProductName=Simscape Electrical
  v^2/R : Fcn  Expr=u^2/r_esr
  v_cap : powerlib/Measurements/Voltage Measurement  PhasorSimulation=off  OutputType=Complex  PSBequivalent=0
      settings: SourceProductName=Simscape Electrical
  v_r : powerlib/Measurements/Voltage Measurement  PhasorSimulation=off  OutputType=Complex  PSBequivalent=0
      settings: SourceProductName=Simscape Electrical
  VCC_in : PMIOPort  Side=Left
  VSS_in : PMIOPort  Port=2  Side=Left
  VCC_out : PMIOPort  Tag=PMCPort  Port=3  Side=Right
  VSS_out : PMIOPort  Tag=PMCPort  Port=4  Side=Right
  v_r_out : Outport
  v_cap_out : Outport  Port=2
  i_leak_out : Outport  Port=3
  p_chg_out : Outport  Port=4
  p_leak_out : Outport  Port=5
  i_out : Outport  Port=6
  c_out : Outport  Port=7
  r_out : Outport  Port=8
  r_leak_out : Outport  Port=9
  l_out : Outport  Port=10
  wires:
  i_leak/1 -> Mux2/1
  v_r/1 -> Mux1/1, v^2/R/1
  Mux6/1 -> c_out/1
  Mux7/1 -> r_out/1
  Mux8/1 -> r_leak_out/1
  Mux9/1 -> l_out/1
  Constant/1 -> Mux6/1
  Constant4/1 -> Mux7/1
  Constant5/1 -> Mux8/1
  ? -> Mux9/1
  c_in/1 -> Mux6/2
  l_in/1 -> Mux9/2
  r_leak_in/1 -> Mux8/2
  r_in/1 -> Mux7/2
  p_chg_in/1 -> Mux3/2
  Mux3/1 -> p_chg_out/1
  v_r_in/1 -> Mux1/2
  Mux1/1 -> v_r_out/1
  v^2/R/1 -> Mux3/1
  Mux2/1 -> i_leak_out/1
  i_leak_in/1 -> Mux2/2
  i/1 -> Mux5/1
  Mux5/1 -> i_out/1
  i_in/1 -> Mux5/2
  p_leak_in/1 -> Mux4/2
  Mux4/1 -> p_leak_out/1
  Mux/1 -> v_cap_out/1
  v_cap_in/1 -> Mux/2
  v_cap/1 -> Fcn1/1, Mux/1
  Fcn1/1 -> Mux4/1
  connections:
  Parallel RLC Branch1/RConn1 -- i_leak/LConn1
  VSS_out/RConn1 -- VSS_in/RConn1 -- i_leak/RConn1 -- Parallel RLC Branch11/RConn1 -- v_cap/LConn2
  v_cap/LConn1 -- Parallel RLC Branch1/LConn1 -- i/RConn1 -- Parallel RLC Branch11/LConn1
  VCC_out/RConn1 -- v_r/LConn1 -- Parallel RLC Branch10/LConn1 -- VCC_in/RConn1
  v_r/LConn2 -- i/LConn1 -- Parallel RLC Branch10/RConn1

== system hybrid_new_eq_circuit_pascal5_single_shot_stack/Supercapacitor 1/Subsystem1/Subsystem1 ==
  note: Export user input data
  v_r_in : Inport
  v_cap_in : Inport  Port=2
  i_leak_in : Inport  Port=3
  p_chg_in : Inport  Port=4
  p_leak_in : Inport  Port=5
  i_in : Inport  Port=6
  c_in : Inport  Port=7
  r_in : Inport  Port=8
  r_leak_in : Inport  Port=9
  l_in : Inport  Port=10
  Constant : Constant  Value=c
  Constant4 : Constant  Value=r_esr
  Constant5 : Constant  Value=r_leak
  Fcn1 : Fcn  Expr=u^2/r_leak
  Mux{,1..9} (10 alike) : Mux  Inputs=2
  Parallel RLC Branch1 : powerlib/Elements/Parallel RLC Branch  LConnTagsString=a  RConnTagsString=__new0  BranchType=R  Resistance=r_leak  Inductance=1e-3  SetiL0=off  InitialCurrent=0  Capacitance=1e-6  Setx0=off  InitialVoltage=0  Measurements=None
      settings: SourceProductName=Simscape Electrical
  Parallel RLC Branch10 : powerlib/Elements/Parallel RLC Branch  LConnTagsString=a  RConnTagsString=__new0  BranchType=R  Resistance=r_esr  Inductance=1e-3  SetiL0=off  InitialCurrent=0  Capacitance=1e-6  Setx0=off  InitialVoltage=0  Measurements=None
      settings: SourceProductName=Simscape Electrical
  Parallel RLC Branch11 : powerlib/Elements/Parallel RLC Branch  LConnTagsString=a  RConnTagsString=__new0  BranchType=C  Resistance=1  Inductance=1e-3  SetiL0=off  InitialCurrent=0  Capacitance=c  Setx0=on  InitialVoltage=v_init  Measurements=None
      settings: SourceProductName=Simscape Electrical
  i : powerlib/Measurements/Current Measurement  PhasorSimulation=off  OutputType=Complex  PSBequivalent=0
      settings: SourceProductName=Simscape Electrical
  i_leak : powerlib/Measurements/Current Measurement  PhasorSimulation=off  OutputType=Complex  PSBequivalent=0
      settings: SourceProductName=Simscape Electrical
  v^2/R : Fcn  Expr=u^2/r_esr
  v_cap : powerlib/Measurements/Voltage Measurement  PhasorSimulation=off  OutputType=Complex  PSBequivalent=0
      settings: SourceProductName=Simscape Electrical
  v_r : powerlib/Measurements/Voltage Measurement  PhasorSimulation=off  OutputType=Complex  PSBequivalent=0
      settings: SourceProductName=Simscape Electrical
  VCC_in : PMIOPort  Side=Left
  VSS_in : PMIOPort  Port=2  Side=Left
  VCC_out : PMIOPort  Tag=PMCPort  Port=3  Side=Right
  VSS_out : PMIOPort  Tag=PMCPort  Port=4  Side=Right
  v_r_out : Outport
  v_cap_out : Outport  Port=2
  i_leak_out : Outport  Port=3
  p_chg_out : Outport  Port=4
  p_leak_out : Outport  Port=5
  i_out : Outport  Port=6
  c_out : Outport  Port=7
  r_out : Outport  Port=8
  r_leak_out : Outport  Port=9
  l_out : Outport  Port=10
  wires:
  i_leak/1 -> Mux2/1
  v_r/1 -> Mux1/1, v^2/R/1
  Mux6/1 -> c_out/1
  Mux7/1 -> r_out/1
  Mux8/1 -> r_leak_out/1
  Mux9/1 -> l_out/1
  Constant/1 -> Mux6/1
  Constant4/1 -> Mux7/1
  Constant5/1 -> Mux8/1
  ? -> Mux9/1
  c_in/1 -> Mux6/2
  l_in/1 -> Mux9/2
  r_leak_in/1 -> Mux8/2
  r_in/1 -> Mux7/2
  p_chg_in/1 -> Mux3/2
  Mux3/1 -> p_chg_out/1
  v_r_in/1 -> Mux1/2
  Mux1/1 -> v_r_out/1
  v^2/R/1 -> Mux3/1
  Mux2/1 -> i_leak_out/1
  i_leak_in/1 -> Mux2/2
  i/1 -> Mux5/1
  Mux5/1 -> i_out/1
  i_in/1 -> Mux5/2
  p_leak_in/1 -> Mux4/2
  Mux4/1 -> p_leak_out/1
  Mux/1 -> v_cap_out/1
  v_cap_in/1 -> Mux/2
  v_cap/1 -> Fcn1/1, Mux/1
  Fcn1/1 -> Mux4/1
  connections:
  Parallel RLC Branch1/RConn1 -- i_leak/LConn1
  VSS_out/RConn1 -- VSS_in/RConn1 -- i_leak/RConn1 -- Parallel RLC Branch11/RConn1 -- v_cap/LConn2
  v_cap/LConn1 -- i/RConn1 -- Parallel RLC Branch11/LConn1 -- Parallel RLC Branch1/LConn1
  VCC_out/RConn1 -- v_r/LConn1 -- Parallel RLC Branch10/LConn1 -- VCC_in/RConn1
  v_r/LConn2 -- i/LConn1 -- Parallel RLC Branch10/RConn1

== system hybrid_new_eq_circuit_pascal5_single_shot_stack/Supercapacitor 1/Subsystem1/Subsystem2 ==
  note: Export user input data
  v_r_in : Inport
  v_cap_in : Inport  Port=2
  i_leak_in : Inport  Port=3
  p_chg_in : Inport  Port=4
  p_leak_in : Inport  Port=5
  i_in : Inport  Port=6
  c_in : Inport  Port=7
  r_in : Inport  Port=8
  r_leak_in : Inport  Port=9
  l_in : Inport  Port=10
  Constant : Constant  Value=c
  Constant4 : Constant  Value=r_esr
  Constant5 : Constant  Value=r_leak
  Fcn1 : Fcn  Expr=u^2/r_leak
  Mux{,1..9} (10 alike) : Mux  Inputs=2
  Parallel RLC Branch1 : powerlib/Elements/Parallel RLC Branch  LConnTagsString=a  RConnTagsString=__new0  BranchType=R  Resistance=r_leak  Inductance=1e-3  SetiL0=off  InitialCurrent=0  Capacitance=1e-6  Setx0=off  InitialVoltage=0  Measurements=None
      settings: SourceProductName=Simscape Electrical
  Parallel RLC Branch10 : powerlib/Elements/Parallel RLC Branch  LConnTagsString=a  RConnTagsString=__new0  BranchType=R  Resistance=r_esr  Inductance=1e-3  SetiL0=off  InitialCurrent=0  Capacitance=1e-6  Setx0=off  InitialVoltage=0  Measurements=None
      settings: SourceProductName=Simscape Electrical
  Parallel RLC Branch11 : powerlib/Elements/Parallel RLC Branch  LConnTagsString=a  RConnTagsString=__new0  BranchType=C  Resistance=1  Inductance=1e-3  SetiL0=off  InitialCurrent=0  Capacitance=c  Setx0=on  InitialVoltage=v_init  Measurements=None
      settings: SourceProductName=Simscape Electrical
  i : powerlib/Measurements/Current Measurement  PhasorSimulation=off  OutputType=Complex  PSBequivalent=0
      settings: SourceProductName=Simscape Electrical
  i_leak : powerlib/Measurements/Current Measurement  PhasorSimulation=off  OutputType=Complex  PSBequivalent=0
      settings: SourceProductName=Simscape Electrical
  v^2/R : Fcn  Expr=u^2/r_esr
  v_cap : powerlib/Measurements/Voltage Measurement  PhasorSimulation=off  OutputType=Complex  PSBequivalent=0
      settings: SourceProductName=Simscape Electrical
  v_r : powerlib/Measurements/Voltage Measurement  PhasorSimulation=off  OutputType=Complex  PSBequivalent=0
      settings: SourceProductName=Simscape Electrical
  VCC_in : PMIOPort  Side=Left
  VSS_in : PMIOPort  Port=2  Side=Left
  VCC_out : PMIOPort  Tag=PMCPort  Port=3  Side=Right
  VSS_out : PMIOPort  Tag=PMCPort  Port=4  Side=Right
  v_r_out : Outport
  v_cap_out : Outport  Port=2
  i_leak_out : Outport  Port=3
  p_chg_out : Outport  Port=4
  p_leak_out : Outport  Port=5
  i_out : Outport  Port=6
  c_out : Outport  Port=7
  r_out : Outport  Port=8
  r_leak_out : Outport  Port=9
  l_out : Outport  Port=10
  wires:
  Fcn1/1 -> Mux4/1
  v_cap/1 -> Mux/1, Fcn1/1
  v_cap_in/1 -> Mux/2
  Mux/1 -> v_cap_out/1
  Mux4/1 -> p_leak_out/1
  p_leak_in/1 -> Mux4/2
  i_in/1 -> Mux5/2
  Mux5/1 -> i_out/1
  i/1 -> Mux5/1
  i_leak_in/1 -> Mux2/2
  Mux2/1 -> i_leak_out/1
  v^2/R/1 -> Mux3/1
  Mux1/1 -> v_r_out/1
  v_r_in/1 -> Mux1/2
  Mux3/1 -> p_chg_out/1
  p_chg_in/1 -> Mux3/2
  r_in/1 -> Mux7/2
  r_leak_in/1 -> Mux8/2
  l_in/1 -> Mux9/2
  c_in/1 -> Mux6/2
  ? -> Mux9/1
  Constant5/1 -> Mux8/1
  Constant4/1 -> Mux7/1
  Constant/1 -> Mux6/1
  Mux9/1 -> l_out/1
  Mux8/1 -> r_leak_out/1
  Mux7/1 -> r_out/1
  Mux6/1 -> c_out/1
  v_r/1 -> v^2/R/1, Mux1/1
  i_leak/1 -> Mux2/1
  connections:
  Parallel RLC Branch10/RConn1 -- i/LConn1 -- v_r/LConn2
  VCC_in/RConn1 -- Parallel RLC Branch10/LConn1 -- v_r/LConn1 -- VCC_out/RConn1
  Parallel RLC Branch1/LConn1 -- Parallel RLC Branch11/LConn1 -- i/RConn1 -- v_cap/LConn1
  v_cap/LConn2 -- Parallel RLC Branch11/RConn1 -- i_leak/RConn1 -- VSS_in/RConn1 -- VSS_out/RConn1
  Parallel RLC Branch1/RConn1 -- i_leak/LConn1

== system hybrid_new_eq_circuit_pascal5_single_shot_stack/Supercapacitor 1/Subsystem1/Subsystem3 ==
  note: Export user input data
  v_r_in : Inport
  v_cap_in : Inport  Port=2
  i_leak_in : Inport  Port=3
  p_chg_in : Inport  Port=4
  p_leak_in : Inport  Port=5
  i_in : Inport  Port=6
  c_in : Inport  Port=7
  r_in : Inport  Port=8
  r_leak_in : Inport  Port=9
  l_in : Inport  Port=10
  Constant : Constant  Value=c
  Constant4 : Constant  Value=r_esr
  Constant5 : Constant  Value=r_leak
  Fcn1 : Fcn  Expr=u^2/r_leak
  Mux{,1..9} (10 alike) : Mux  Inputs=2
  Parallel RLC Branch1 : powerlib/Elements/Parallel RLC Branch  LConnTagsString=a  RConnTagsString=__new0  BranchType=R  Resistance=r_leak  Inductance=1e-3  SetiL0=off  InitialCurrent=0  Capacitance=1e-6  Setx0=off  InitialVoltage=0  Measurements=None
      settings: SourceProductName=Simscape Electrical
  Parallel RLC Branch10 : powerlib/Elements/Parallel RLC Branch  LConnTagsString=a  RConnTagsString=__new0  BranchType=R  Resistance=r_esr  Inductance=1e-3  SetiL0=off  InitialCurrent=0  Capacitance=1e-6  Setx0=off  InitialVoltage=0  Measurements=None
      settings: SourceProductName=Simscape Electrical
  Parallel RLC Branch11 : powerlib/Elements/Parallel RLC Branch  LConnTagsString=a  RConnTagsString=__new0  BranchType=C  Resistance=1  Inductance=1e-3  SetiL0=off  InitialCurrent=0  Capacitance=c  Setx0=on  InitialVoltage=v_init  Measurements=None
      settings: SourceProductName=Simscape Electrical
  i : powerlib/Measurements/Current Measurement  PhasorSimulation=off  OutputType=Complex  PSBequivalent=0
      settings: SourceProductName=Simscape Electrical
  i_leak : powerlib/Measurements/Current Measurement  PhasorSimulation=off  OutputType=Complex  PSBequivalent=0
      settings: SourceProductName=Simscape Electrical
  v^2/R : Fcn  Expr=u^2/r_esr
  v_cap : powerlib/Measurements/Voltage Measurement  PhasorSimulation=off  OutputType=Complex  PSBequivalent=0
      settings: SourceProductName=Simscape Electrical
  v_r : powerlib/Measurements/Voltage Measurement  PhasorSimulation=off  OutputType=Complex  PSBequivalent=0
      settings: SourceProductName=Simscape Electrical
  VCC_in : PMIOPort  Side=Left
  VSS_in : PMIOPort  Port=2  Side=Left
  VCC_out : PMIOPort  Tag=PMCPort  Port=3  Side=Right
  VSS_out : PMIOPort  Tag=PMCPort  Port=4  Side=Right
  v_r_out : Outport
  v_cap_out : Outport  Port=2
  i_leak_out : Outport  Port=3
  p_chg_out : Outport  Port=4
  p_leak_out : Outport  Port=5
  i_out : Outport  Port=6
  c_out : Outport  Port=7
  r_out : Outport  Port=8
  r_leak_out : Outport  Port=9
  l_out : Outport  Port=10
  wires:
  i_leak/1 -> Mux2/1
  v_r/1 -> Mux1/1, v^2/R/1
  Mux6/1 -> c_out/1
  Mux7/1 -> r_out/1
  Mux8/1 -> r_leak_out/1
  Mux9/1 -> l_out/1
  Constant/1 -> Mux6/1
  Constant4/1 -> Mux7/1
  Constant5/1 -> Mux8/1
  ? -> Mux9/1
  c_in/1 -> Mux6/2
  l_in/1 -> Mux9/2
  r_leak_in/1 -> Mux8/2
  r_in/1 -> Mux7/2
  p_chg_in/1 -> Mux3/2
  Mux3/1 -> p_chg_out/1
  v_r_in/1 -> Mux1/2
  Mux1/1 -> v_r_out/1
  v^2/R/1 -> Mux3/1
  Mux2/1 -> i_leak_out/1
  i_leak_in/1 -> Mux2/2
  i/1 -> Mux5/1
  Mux5/1 -> i_out/1
  i_in/1 -> Mux5/2
  p_leak_in/1 -> Mux4/2
  Mux4/1 -> p_leak_out/1
  Mux/1 -> v_cap_out/1
  v_cap_in/1 -> Mux/2
  v_cap/1 -> Fcn1/1, Mux/1
  Fcn1/1 -> Mux4/1
  connections:
  Parallel RLC Branch1/RConn1 -- i_leak/LConn1
  VSS_out/RConn1 -- VSS_in/RConn1 -- i_leak/RConn1 -- Parallel RLC Branch11/RConn1 -- v_cap/LConn2
  v_cap/LConn1 -- i/RConn1 -- Parallel RLC Branch11/LConn1 -- Parallel RLC Branch1/LConn1
  VCC_out/RConn1 -- v_r/LConn1 -- Parallel RLC Branch10/LConn1 -- VCC_in/RConn1
  v_r/LConn2 -- i/LConn1 -- Parallel RLC Branch10/RConn1
